simulink model "app_logic"  (R2025a)
settings: Solver=VariableStepAuto  StartTime=0.0  StopTime=inf  RelTol=1e-3
libraries: instrumentseriallib x3, dspstat3 x1
settings Model: Creator=Athaariq  LastModifiedBy=Athaariq

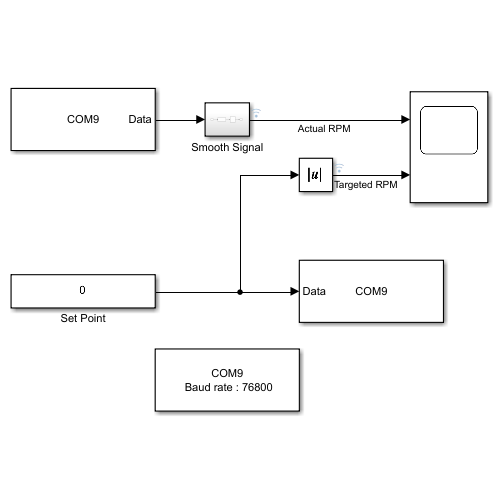
[thumbnail: Simulink's stored preview of the top-level diagram]
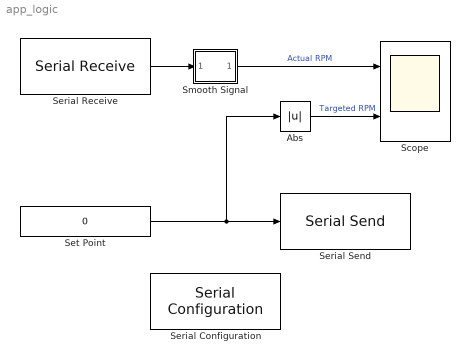
== system app_logic ==
  Abs : Abs  SaturateOnIntegerOverflow=off
  Scope : Scope  NumInputPorts=2
      settings: ActiveDisplayYMinimum=-1  ActiveDisplayYMaximum=1
  Serial Configuration : instrumentseriallib/Serial Configuration  Priority=-200000  PortSel=COM9  Port=COM9  ComPort=COM9  BaudRate=76800  DataBits=8  Parity=none  StopBits=1  ByteOrder=little-endian  FlowControl=none  Timeout=10  SimulateUsing=Interpreted execution  BlockInModel=on  aMode=1
  Serial Receive : instrumentseriallib/Serial Receive  Priority=1  PortSel=COM9  Port=COM9  ComPort=COM9  DataType=uint16  SaveDataType=uint8  ToggleHeader=off  Header=[165 165]  ToggleDataSize=on  DataSize=[1 1]  ToggleTerminator=off  Terminator=Custom terminator  CustomTerminator=[90 90]  InputFormat=Column major  EnableBlockingMode=on  ActionDataUnavailable=Output last received value  ActionWhenDataUnavailable=Output last received value  CustomValue=0  SampleTime=0.01  SimulateUsing=Interpreted execution  BlockInModel=on  aMode=1  LibraryInUse=instrumentlib
  Serial Send : instrumentseriallib/Serial Send  Priority=1  PortSel=COM9  Port=COM9  ComPort=COM9  Header=[]  Terminator=<none>  CustomTerminator=[90 90]  EnableBlockingMode=on  SimulateUsing=Interpreted execution  BlockInModel=on  aMode=1
  Set Point : Constant  Value=0  OutDataTypeStr=int16  SampleTime=-1  LockScale=on
  Smooth Signal : Subsystem
  wires:
  Serial Receive/1 -> Smooth Signal/1(Raw RPM)
  Abs/1 -> Scope/2  "Targeted RPM"
  Set Point/1 -> Abs/1, Serial Send/1
  Smooth Signal/1(Measured RPM) -> Scope/1  "Actual RPM"

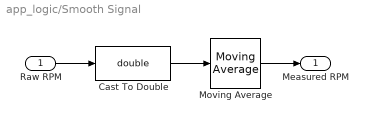
== system app_logic/Smooth Signal ==
  Raw RPM : Inport
  Cast To Double : DataTypeConversion  OutDataTypeStr=double  SaturateOnIntegerOverflow=off  RndMeth=Floor
  Moving Average : dspstat3/Moving Average  Method=Sliding window  ForgettingFactorPort=off  SpecifyWindowLength=on  WindowLength=10  OverlapLength=9  AllowArbitraryInputLength=off  ForgettingFactor=0.8  SimulateUsing=Code generation
  Measured RPM : Outport
  wires:
  Raw RPM/1 -> Cast To Double/1
  Moving Average/1 -> Measured RPM/1
  Cast To Double/1 -> Moving Average/1
